simulink model "FM_04_Desacoplado_Simplificado"  (Simulink 7.1)
settings: Solver=ode45  StartTime=0.0  StopTime=300  RelTol=1e-3
undefined symbols (not defined in the file or in its folder): analoginput, analogoutput, QT
libraries: daqlib x2, simulink x2, simulink_extras x2
settings Model: Creator=didaticontrol  LastModifiedBy=didaticontrol

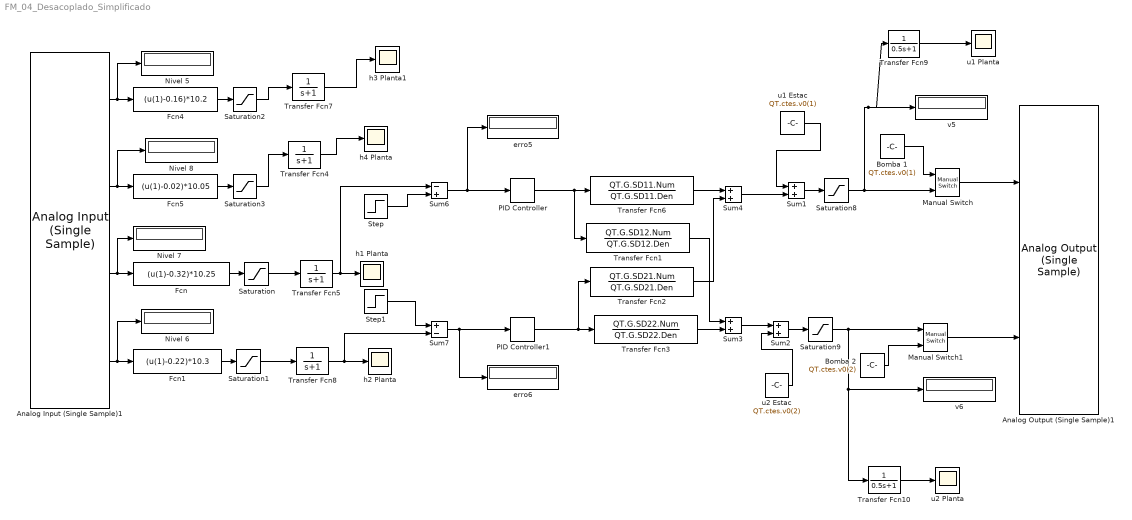
== system FM_04_Desacoplado_Simplificado ==
  Analog Input (Single Sample)1 : daqlib/Analog Input (Single Sample)  DialogController=daqcreatedialog  DialogControllerArgs=DataTag0  DeviceMenu=nidaq Dev1 (USB-6008)  Device=nidaq Dev1 (USB-6008)  ObjConstructor=analoginput('nidaq','Dev1')  InputType=Differential  NChannelsSelected=4  Channels=1$0$$5$#1$1$$5$#1$2$$5$#1$3$$5$#  NPorts=1 per hardware channel  BlockSampleTime=10e-3
  Analog Output (Single Sample)1 : daqlib/Analog Output (Single Sample)  DialogController=daqcreatedialog  DialogControllerArgs=DataTag1  DeviceMenu=nidaq Dev1 (USB-6008)  Device=nidaq Dev1 (USB-6008)  ObjConstructor=analogoutput('nidaq','Dev1')  NChannelsSelected=2  Channels=1$0$$1$0$#1$1$$1$0$#  NPorts=1 per hardware channel
  Bomba 1 : Constant  Value=QT.ctes.v0(1)
  Bomba 2 : Constant  Value=QT.ctes.v0(2)
  Fcn : Fcn  Expr=(u(1)-0.32)*10.25  SampleTime=10e-3
  Fcn1 : Fcn  Expr=(u(1)-0.22)*10.3
  Fcn4 : Fcn  Expr=(u(1)-0.16)*10.2
  Fcn5 : Fcn  Expr=(u(1)-0.02)*10.05
  Manual Switch : simulink/Signal Routing/Manual Switch  SystemSampleTime=-1  sw=1  action=0  varsize=off
  Manual Switch1 : simulink/Signal Routing/Manual Switch  SystemSampleTime=-1  sw=0  action=0  varsize=off
  Nivel {5..8} (4 alike) : Display
  PID Controller : simulink_extras/Additional Linear/PID Controller  SystemSampleTime=-1  P=7  I=0.2  D=0
  PID Controller1 : simulink_extras/Additional Linear/PID Controller  SystemSampleTime=-1  P=4  I=0.2  D=0
  Saturation : Saturate  UpperLimit=23  LowerLimit=0  SampleTime=10e-3
  Saturation1 : Saturate  UpperLimit=23  LowerLimit=0
  Saturation2 : Saturate  UpperLimit=23  LowerLimit=0
  Saturation3 : Saturate  UpperLimit=23  LowerLimit=0
  Saturation8 : Saturate  UpperLimit=0.7*5  LowerLimit=0  SampleTime=10e-3
  Saturation9 : Saturate  UpperLimit=0.7*5  LowerLimit=0  SampleTime=10e-3
  Step : Step  Time=100  Before=QT.ctes.h0(1)  After=QT.ctes.h0(1)+1  SampleTime=0
  Step1 : Step  Time=200  Before=QT.ctes.h0(2)  After=QT.ctes.h0(2)+1  SampleTime=0
  Sum{1..4} (4 alike) : Sum  OutDataType=sfix(16)  OutScaling=2^0
  Sum6 : Sum  Inputs=-+  OutDataType=sfix(16)  OutScaling=2^0
  Sum7 : Sum  Inputs=+-  OutDataType=sfix(16)  OutScaling=2^0
  Transfer Fcn1 : TransferFcn  Numerator=QT.G.SD12.Num  Denominator=QT.G.SD12.Den
  Transfer Fcn10 : TransferFcn  Denominator=[0.5 1]
  Transfer Fcn2 : TransferFcn  Numerator=QT.G.SD21.Num  Denominator=QT.G.SD21.Den
  Transfer Fcn3 : TransferFcn  Numerator=QT.G.SD22.Num  Denominator=QT.G.SD22.Den
  Transfer Fcn{4..5,7..8} (4 alike) : TransferFcn  Denominator=[1 1]
  Transfer Fcn6 : TransferFcn  Numerator=QT.G.SD11.Num  Denominator=QT.G.SD11.Den
  Transfer Fcn9 : TransferFcn  Denominator=[0.5 1]
  erro5 : Display
  erro6 : Display
  h1 Planta : Scope
      settings: YMin=0  YMax=8.5  SaveName=h1_real
  h2 Planta : Scope
      settings: TimeRange=300  YMin=0  YMax=11  SaveName=h2_real
  h3 Planta1 : Scope
      settings: YMin=0  YMax=8.5  SaveName=h3_real
  h4 Planta : Scope
      settings: YMin=0  YMax=15  SaveName=h4_real
  u1 Planta : Scope
      settings: YMin=1.75  YMax=3.5  SaveName=u1_real
  u1 Estac : Constant  Value=QT.ctes.v0(1)
  u2 Planta : Scope
      settings: YMin=9.2  YMax=10.2  SaveName=u2_real
  u2 Estac : Constant  Value=QT.ctes.v0(2)
  v5 : Display
  v6 : Display
  wires:
  Analog Input (Single Sample)1/3 -> Fcn/1, Nivel 7/1
  Fcn/1 -> Saturation/1
  Fcn1/1 -> Saturation1/1
  Analog Input (Single Sample)1/4 -> Fcn1/1, Nivel 6/1
  Saturation/1 -> Transfer Fcn5/1
  Analog Input (Single Sample)1/2 -> Fcn5/1, Nivel 8/1
  Analog Input (Single Sample)1/1 -> Nivel 5/1, Fcn4/1
  Fcn4/1 -> Saturation2/1
  Fcn5/1 -> Saturation3/1
  Manual Switch/1 -> Analog Output (Single Sample)1/1
  Manual Switch1/1 -> Analog Output (Single Sample)1/2
  Bomba 1/1 -> Manual Switch/1
  Sum6/1 -> erro5/1, PID Controller/1
  Sum7/1 -> erro6/1, PID Controller1/1
  Saturation8/1 -> Manual Switch/2, v5/1, Transfer Fcn9/1
  Saturation9/1 -> Manual Switch1/1, v6/1, Transfer Fcn10/1
  Bomba 2/1 -> Manual Switch1/2
  Saturation1/1 -> Transfer Fcn8/1
  Step/1 -> Sum6/2
  Step1/1 -> Sum7/1
  Sum1/1 -> Saturation8/1
  PID Controller/1 -> Transfer Fcn1/1, Transfer Fcn6/1
  u1 Estac/1 -> Sum1/1
  Sum2/1 -> Saturation9/1
  u2 Estac/1 -> Sum2/2
  Sum4/1 -> Sum1/2
  Transfer Fcn2/1 -> Sum4/2
  Sum3/1 -> Sum2/1
  Transfer Fcn1/1 -> Sum3/1
  Transfer Fcn3/1 -> Sum3/2
  Transfer Fcn6/1 -> Sum4/1
  PID Controller1/1 -> Transfer Fcn2/1, Transfer Fcn3/1
  Transfer Fcn7/1 -> h3 Planta1/1
  Saturation2/1 -> Transfer Fcn7/1
  Saturation3/1 -> Transfer Fcn4/1
  Transfer Fcn4/1 -> h4 Planta/1
  Transfer Fcn5/1 -> h1 Planta/1, Sum6/1
  Transfer Fcn8/1 -> h2 Planta/1, Sum7/2
  Transfer Fcn9/1 -> u1 Planta/1
  Transfer Fcn10/1 -> u2 Planta/1
